simulink model "Hopf_AXILite"  (R2020a)
settings: Solver=VariableStepAuto  StartTime=0.0  StopTime=500  RelTol=1e-3
undefined symbols (not defined in the file): AXI4, Lite
libraries: xbsIndex_r4 x256
(part 2 of 2)

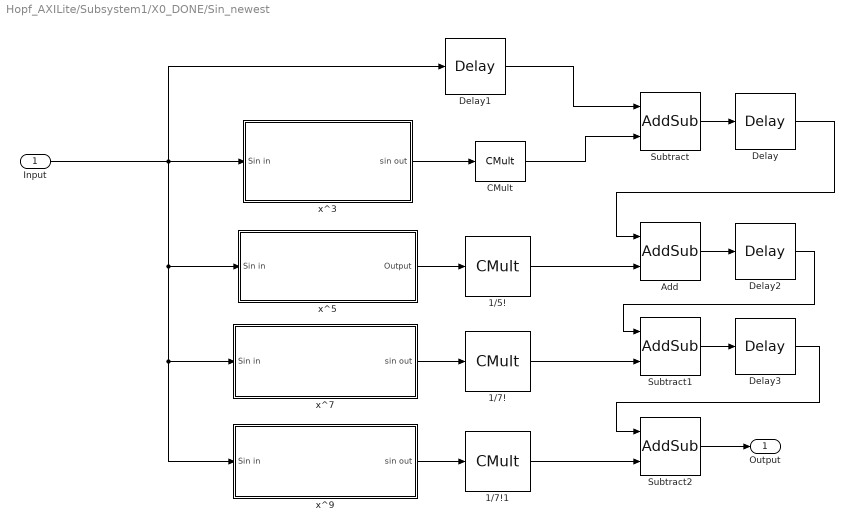
== system Hopf_AXILite/Subsystem1/X0_DONE/Sin_newest ==
  "Input " : Inport
  1/5! : xbsIndex_r4/CMult  const=1/(1*2*3*4*5)  gui_display_data_type=Fixed-point  const_n_bits=24  const_bin_pt=18  float_type=Single  exp_bits=8  fraction_bits=24  en=off  latency=1  precision=User Defined  arith_type="Signed  (2's comp)"  n_bits=24  bin_pt=18  quantization=Truncate  overflow=Wrap  use_behavioral_HDL=off  mem_type=Distributed RAM  pipeline=off  dbl_ovrd=off  block_type=cmult
  1/7! : xbsIndex_r4/CMult  const=1/(1*2*3*4*5*6*7)  gui_display_data_type=Fixed-point  const_n_bits=24  const_bin_pt=18  float_type=Single  exp_bits=8  fraction_bits=24  en=off  latency=1  precision=User Defined  arith_type="Signed  (2's comp)"  n_bits=24  bin_pt=18  quantization=Truncate  overflow=Wrap  use_behavioral_HDL=off  mem_type=Distributed RAM  pipeline=off  dbl_ovrd=off  block_type=cmult
  1/7!1 : xbsIndex_r4/CMult  const=1/(1*2*3*4*5*6*7*8*9)  gui_display_data_type=Fixed-point  const_n_bits=24  const_bin_pt=18  float_type=Single  exp_bits=8  fraction_bits=24  en=off  latency=1  precision=User Defined  arith_type="Signed  (2's comp)"  n_bits=24  bin_pt=18  quantization=Truncate  overflow=Wrap  use_behavioral_HDL=off  mem_type=Distributed RAM  pipeline=off  dbl_ovrd=off  block_type=cmult
  Add : xbsIndex_r4/AddSub  mode=Addition  use_carryin=off  use_carryout=off  en=off  latency=1  precision=User Defined  arith_type=Unsigned  n_bits=24  bin_pt=18  quantization=Truncate  overflow=Wrap  use_behavioral_HDL=off  hw_selection=Fabric  pipelined=off  dbl_ovrd=off  block_type=addsub
  CMult : xbsIndex_r4/CMult  const=1/2  gui_display_data_type=Fixed-point  const_n_bits=24  const_bin_pt=18  float_type=Single  exp_bits=8  fraction_bits=24  en=off  latency=1  precision=User Defined  arith_type="Signed  (2's comp)"  n_bits=24  bin_pt=19  quantization=Truncate  overflow=Wrap  use_behavioral_HDL=off  mem_type=Distributed RAM  pipeline=off  dbl_ovrd=off  block_type=cmult
  Delay : xbsIndex_r4/Delay  rst=off  infoeditControl=Selection of Reset will increase slice count due to use of real FFs and instead of SRLs  en=off  latency=2  reg_retiming=off  dbl_ovrd=off  block_type=delay
  Delay1 : xbsIndex_r4/Delay  rst=off  infoeditControl=Selection of Reset will increase slice count due to use of real FFs and instead of SRLs  en=off  latency=7  reg_retiming=off  dbl_ovrd=off  block_type=delay
  Delay2 : xbsIndex_r4/Delay  rst=off  infoeditControl=Selection of Reset will increase slice count due to use of real FFs and instead of SRLs  en=off  latency=2  reg_retiming=off  dbl_ovrd=off  block_type=delay
  Delay3 : xbsIndex_r4/Delay  rst=off  infoeditControl=Selection of Reset will increase slice count due to use of real FFs and instead of SRLs  en=off  latency=2  reg_retiming=off  dbl_ovrd=off  block_type=delay
  Subtract : xbsIndex_r4/AddSub  mode=Subtraction  use_carryin=off  use_carryout=off  en=off  latency=1  precision=User Defined  arith_type=Unsigned  n_bits=24  bin_pt=18  quantization=Truncate  overflow=Wrap  use_behavioral_HDL=off  hw_selection=Fabric  pipelined=off  dbl_ovrd=off  block_type=addsub
  Subtract1 : xbsIndex_r4/AddSub  mode=Subtraction  use_carryin=off  use_carryout=off  en=off  latency=1  precision=User Defined  arith_type=Unsigned  n_bits=24  bin_pt=18  quantization=Truncate  overflow=Wrap  use_behavioral_HDL=off  hw_selection=Fabric  pipelined=off  dbl_ovrd=off  block_type=addsub
  Subtract2 : xbsIndex_r4/AddSub  mode=Addition  use_carryin=off  use_carryout=off  en=off  latency=1  precision=User Defined  arith_type=Unsigned  n_bits=24  bin_pt=18  quantization=Truncate  overflow=Wrap  use_behavioral_HDL=off  hw_selection=Fabric  pipelined=off  dbl_ovrd=off  block_type=addsub
  x^3 : Subsystem
  x^5 : Subsystem
  x^7 : Subsystem
  x^9 : Subsystem
  Output : Outport
  wires:
  Add/1 -> Delay2/1
  Subtract1/1 -> Delay3/1
  1/5!/1 -> Add/2
  1/7!/1 -> Subtract1/2
  Delay1/1 -> Subtract/1
  "Input "/1 -> Delay1/1, x^3/1(Sin in), x^9/1(Sin in), x^7/1(Sin in), x^5/1(Sin in)
  x^3/1(sin out) -> CMult/1
  x^5/1(Output) -> 1/5!/1
  x^7/1(sin out) -> 1/7!/1
  Subtract/1 -> Delay/1
  Delay2/1 -> Subtract1/1
  x^9/1(sin out) -> 1/7!1/1
  Delay3/1 -> Subtract2/1
  1/7!1/1 -> Subtract2/2
  Subtract2/1 -> Output/1
  Delay/1 -> Add/1
  CMult/1 -> Subtract/2

== system Hopf_AXILite/Subsystem1/Calculation x1/Sin_newest/x^3 ==
  Sin in : Inport
  Mult2 : xbsIndex_r4/Mult  precision=User Defined  arith_type="Signed  (2's comp)"  n_bits=24  bin_pt=18  quantization=Truncate  overflow=Wrap  en=off  latency=3  use_behavioral_HDL=off  opt=Speed  use_embedded=on  optimum_pipeline=off  pipeline=on  dbl_ovrd=off  use_rpm=on  placement_style=Triangular  block_type=mult
  Mult3 : xbsIndex_r4/Mult  precision=User Defined  arith_type="Signed  (2's comp)"  n_bits=24  bin_pt=18  quantization=Truncate  overflow=Wrap  en=off  latency=3  use_behavioral_HDL=off  opt=Speed  use_embedded=on  optimum_pipeline=off  pipeline=on  dbl_ovrd=off  use_rpm=on  placement_style=Triangular  block_type=mult
  sin out : Outport
  wires:
  Mult2/1 -> Mult3/1
  Sin in/1 -> Mult2/1, Mult3/2, Mult2/2
  Mult3/1 -> sin out/1

== system Hopf_AXILite/Subsystem1/Calculation x1/Sin_newest/x^5 ==
  Sin in : Inport
  Mult2 : xbsIndex_r4/Mult  precision=User Defined  arith_type="Signed  (2's comp)"  n_bits=24  bin_pt=18  quantization=Truncate  overflow=Wrap  en=off  latency=3  use_behavioral_HDL=off  opt=Speed  use_embedded=on  optimum_pipeline=off  pipeline=on  dbl_ovrd=off  use_rpm=on  placement_style=Triangular  block_type=mult
  Mult3 : xbsIndex_r4/Mult  precision=User Defined  arith_type="Signed  (2's comp)"  n_bits=24  bin_pt=18  quantization=Truncate  overflow=Wrap  en=off  latency=3  use_behavioral_HDL=off  opt=Speed  use_embedded=on  optimum_pipeline=off  pipeline=on  dbl_ovrd=off  use_rpm=on  placement_style=Triangular  block_type=mult
  Mult4 : xbsIndex_r4/Mult  precision=User Defined  arith_type="Signed  (2's comp)"  n_bits=24  bin_pt=18  quantization=Truncate  overflow=Wrap  en=off  latency=3  use_behavioral_HDL=off  opt=Speed  use_embedded=on  optimum_pipeline=off  pipeline=on  dbl_ovrd=off  use_rpm=on  placement_style=Triangular  block_type=mult
  Output : Outport
  wires:
  Mult3/1 -> Mult4/1, Mult4/2
  Mult2/1 -> Mult3/1
  Sin in/1 -> Mult2/1, Mult3/2, Mult2/2
  Mult4/1 -> Output/1

== system Hopf_AXILite/Subsystem1/Calculation x1/Sin_newest/x^7 ==
  Sin in : Inport
  Mult{1..4} (4 alike) : xbsIndex_r4/Mult  precision=User Defined  arith_type="Signed  (2's comp)"  n_bits=24  bin_pt=18  quantization=Truncate  overflow=Wrap  en=off  latency=3  use_behavioral_HDL=off  opt=Speed  use_embedded=on  optimum_pipeline=off  pipeline=on  dbl_ovrd=off  use_rpm=on  placement_style=Triangular  block_type=mult
  sin out : Outport
  wires:
  Mult2/1 -> Mult3/1
  Mult3/1 -> Mult4/1, Mult4/2
  Mult4/1 -> Mult1/2, Mult1/1
  Sin in/1 -> Mult3/2, Mult2/2, Mult2/1
  Mult1/1 -> sin out/1

== system Hopf_AXILite/Subsystem1/Calculation x1/Sin_newest/x^9 ==
  Sin in : Inport
  Mult{1..5} (5 alike) : xbsIndex_r4/Mult  precision=User Defined  arith_type="Signed  (2's comp)"  n_bits=24  bin_pt=18  quantization=Truncate  overflow=Wrap  en=off  latency=3  use_behavioral_HDL=off  opt=Speed  use_embedded=on  optimum_pipeline=off  pipeline=on  dbl_ovrd=off  use_rpm=on  placement_style=Triangular  block_type=mult
  sin out : Outport
  wires:
  Mult2/1 -> Mult3/1
  Mult3/1 -> Mult4/1, Mult4/2
  Mult4/1 -> Mult1/2, Mult1/1
  Sin in/1 -> Mult3/2, Mult2/2, Mult2/1
  Mult1/1 -> Mult5/1, Mult5/2
  Mult5/1 -> sin out/1

== system Hopf_AXILite/Subsystem1/Calculation x1/Sin_newest1/x^3 ==
  Sin in : Inport
  Mult2 : xbsIndex_r4/Mult  precision=User Defined  arith_type="Signed  (2's comp)"  n_bits=24  bin_pt=18  quantization=Truncate  overflow=Wrap  en=off  latency=3  use_behavioral_HDL=off  opt=Speed  use_embedded=on  optimum_pipeline=off  pipeline=on  dbl_ovrd=off  use_rpm=on  placement_style=Triangular  block_type=mult
  Mult3 : xbsIndex_r4/Mult  precision=User Defined  arith_type="Signed  (2's comp)"  n_bits=24  bin_pt=18  quantization=Truncate  overflow=Wrap  en=off  latency=3  use_behavioral_HDL=off  opt=Speed  use_embedded=on  optimum_pipeline=off  pipeline=on  dbl_ovrd=off  use_rpm=on  placement_style=Triangular  block_type=mult
  sin out : Outport
  wires:
  Mult2/1 -> Mult3/1
  Sin in/1 -> Mult2/1, Mult3/2, Mult2/2
  Mult3/1 -> sin out/1

== system Hopf_AXILite/Subsystem1/Calculation x1/Sin_newest1/x^5 ==
  Sin in : Inport
  Mult2 : xbsIndex_r4/Mult  precision=User Defined  arith_type="Signed  (2's comp)"  n_bits=24  bin_pt=18  quantization=Truncate  overflow=Wrap  en=off  latency=3  use_behavioral_HDL=off  opt=Speed  use_embedded=on  optimum_pipeline=off  pipeline=on  dbl_ovrd=off  use_rpm=on  placement_style=Triangular  block_type=mult
  Mult3 : xbsIndex_r4/Mult  precision=User Defined  arith_type="Signed  (2's comp)"  n_bits=24  bin_pt=18  quantization=Truncate  overflow=Wrap  en=off  latency=3  use_behavioral_HDL=off  opt=Speed  use_embedded=on  optimum_pipeline=off  pipeline=on  dbl_ovrd=off  use_rpm=on  placement_style=Triangular  block_type=mult
  Mult4 : xbsIndex_r4/Mult  precision=User Defined  arith_type="Signed  (2's comp)"  n_bits=24  bin_pt=18  quantization=Truncate  overflow=Wrap  en=off  latency=3  use_behavioral_HDL=off  opt=Speed  use_embedded=on  optimum_pipeline=off  pipeline=on  dbl_ovrd=off  use_rpm=on  placement_style=Triangular  block_type=mult
  Output : Outport
  wires:
  Mult3/1 -> Mult4/1, Mult4/2
  Mult2/1 -> Mult3/1
  Sin in/1 -> Mult2/1, Mult3/2, Mult2/2
  Mult4/1 -> Output/1

== system Hopf_AXILite/Subsystem1/Calculation x1/Sin_newest1/x^7 ==
  Sin in : Inport
  Mult{1..4} (4 alike) : xbsIndex_r4/Mult  precision=User Defined  arith_type="Signed  (2's comp)"  n_bits=24  bin_pt=18  quantization=Truncate  overflow=Wrap  en=off  latency=3  use_behavioral_HDL=off  opt=Speed  use_embedded=on  optimum_pipeline=off  pipeline=on  dbl_ovrd=off  use_rpm=on  placement_style=Triangular  block_type=mult
  sin out : Outport
  wires:
  Mult2/1 -> Mult3/1
  Mult3/1 -> Mult4/1, Mult4/2
  Mult4/1 -> Mult1/2, Mult1/1
  Sin in/1 -> Mult3/2, Mult2/2, Mult2/1
  Mult1/1 -> sin out/1

== system Hopf_AXILite/Subsystem1/Calculation x1/Sin_newest1/x^9 ==
  Sin in : Inport
  Mult{1..5} (5 alike) : xbsIndex_r4/Mult  precision=User Defined  arith_type="Signed  (2's comp)"  n_bits=24  bin_pt=18  quantization=Truncate  overflow=Wrap  en=off  latency=3  use_behavioral_HDL=off  opt=Speed  use_embedded=on  optimum_pipeline=off  pipeline=on  dbl_ovrd=off  use_rpm=on  placement_style=Triangular  block_type=mult
  sin out : Outport
  wires:
  Mult2/1 -> Mult3/1
  Mult3/1 -> Mult4/1, Mult4/2
  Mult4/1 -> Mult1/2, Mult1/1
  Sin in/1 -> Mult3/2, Mult2/2, Mult2/1
  Mult1/1 -> Mult5/1, Mult5/2
  Mult5/1 -> sin out/1

== system Hopf_AXILite/Subsystem1/Calculation x2/Cosine_newest/POW 10 ==
  Input : Inport
  Mult{1..5} (5 alike) : xbsIndex_r4/Mult  precision=User Defined  arith_type="Signed  (2's comp)"  n_bits=24  bin_pt=18  quantization=Truncate  overflow=Wrap  en=off  latency=3  use_behavioral_HDL=off  opt=Speed  use_embedded=on  optimum_pipeline=off  pipeline=on  dbl_ovrd=off  use_rpm=on  placement_style=Triangular  block_type=mult
  ^10 : Outport
  wires:
  Mult2/1 -> Mult1/1, Mult1/2
  Mult1/1 -> Mult3/1, Mult3/2
  Mult3/1 -> Mult4/1, Mult4/2
  Mult4/1 -> Mult5/1, Mult5/2
  Input/1 -> Mult2/1, Mult2/2
  Mult5/1 -> ^10/1

== system Hopf_AXILite/Subsystem1/Calculation x2/Cosine_newest/POW 8 ==
  Input : Inport
  Mult{1..4} (4 alike) : xbsIndex_r4/Mult  precision=User Defined  arith_type="Signed  (2's comp)"  n_bits=24  bin_pt=18  quantization=Truncate  overflow=Wrap  en=off  latency=3  use_behavioral_HDL=off  opt=Speed  use_embedded=on  optimum_pipeline=off  pipeline=on  dbl_ovrd=off  use_rpm=on  placement_style=Triangular  block_type=mult
  ^8 : Outport
  wires:
  Mult2/1 -> Mult1/1, Mult1/2
  Mult1/1 -> Mult3/1, Mult3/2
  Mult3/1 -> Mult4/1, Mult4/2
  Input/1 -> Mult2/1, Mult2/2
  Mult4/1 -> ^8/1

== system Hopf_AXILite/Subsystem1/Calculation x2/Cosine_newest/Subsystem ==
  Input : Inport
  Mult1 : xbsIndex_r4/Mult  precision=User Defined  arith_type="Signed  (2's comp)"  n_bits=24  bin_pt=18  quantization=Truncate  overflow=Wrap  en=off  latency=3  use_behavioral_HDL=off  opt=Speed  use_embedded=on  optimum_pipeline=off  pipeline=on  dbl_ovrd=off  use_rpm=on  placement_style=Triangular  block_type=mult
  Mult2 : xbsIndex_r4/Mult  precision=User Defined  arith_type="Signed  (2's comp)"  n_bits=24  bin_pt=18  quantization=Truncate  overflow=Wrap  en=off  latency=3  use_behavioral_HDL=off  opt=Speed  use_embedded=on  optimum_pipeline=off  pipeline=on  dbl_ovrd=off  use_rpm=on  placement_style=Triangular  block_type=mult
  ^4 : Outport
  wires:
  Mult2/1 -> Mult1/2, Mult1/1
  Input/1 -> Mult2/2, Mult2/1
  Mult1/1 -> ^4/1

== system Hopf_AXILite/Subsystem1/Calculation x2/Cosine_newest/Subsystem1 ==
  Input : Inport
  Mult1 : xbsIndex_r4/Mult  precision=User Defined  arith_type="Signed  (2's comp)"  n_bits=24  bin_pt=18  quantization=Truncate  overflow=Wrap  en=off  latency=3  use_behavioral_HDL=off  opt=Speed  use_embedded=on  optimum_pipeline=off  pipeline=on  dbl_ovrd=off  use_rpm=on  placement_style=Triangular  block_type=mult
  Mult2 : xbsIndex_r4/Mult  precision=User Defined  arith_type="Signed  (2's comp)"  n_bits=24  bin_pt=18  quantization=Truncate  overflow=Wrap  en=off  latency=3  use_behavioral_HDL=off  opt=Speed  use_embedded=on  optimum_pipeline=off  pipeline=on  dbl_ovrd=off  use_rpm=on  placement_style=Triangular  block_type=mult
  Mult3 : xbsIndex_r4/Mult  precision=User Defined  arith_type="Signed  (2's comp)"  n_bits=24  bin_pt=18  quantization=Truncate  overflow=Wrap  en=off  latency=3  use_behavioral_HDL=off  opt=Speed  use_embedded=on  optimum_pipeline=off  pipeline=on  dbl_ovrd=off  use_rpm=on  placement_style=Triangular  block_type=mult
  ^6 : Outport
  wires:
  Mult2/1 -> Mult1/2, Mult1/1
  Mult1/1 -> Mult3/2, Mult3/1
  Input/1 -> Mult2/2, Mult2/1
  Mult3/1 -> ^6/1

== system Hopf_AXILite/Subsystem1/Calculation x2/Cosine_newest1/POW 10 ==
  Input : Inport
  Mult{1..5} (5 alike) : xbsIndex_r4/Mult  precision=User Defined  arith_type="Signed  (2's comp)"  n_bits=24  bin_pt=18  quantization=Truncate  overflow=Wrap  en=off  latency=3  use_behavioral_HDL=off  opt=Speed  use_embedded=on  optimum_pipeline=off  pipeline=on  dbl_ovrd=off  use_rpm=on  placement_style=Triangular  block_type=mult
  ^10 : Outport
  wires:
  Mult2/1 -> Mult1/1, Mult1/2
  Mult1/1 -> Mult3/1, Mult3/2
  Mult3/1 -> Mult4/1, Mult4/2
  Mult4/1 -> Mult5/1, Mult5/2
  Input/1 -> Mult2/1, Mult2/2
  Mult5/1 -> ^10/1

== system Hopf_AXILite/Subsystem1/Calculation x2/Cosine_newest1/POW 8 ==
  Input : Inport
  Mult{1..4} (4 alike) : xbsIndex_r4/Mult  precision=User Defined  arith_type="Signed  (2's comp)"  n_bits=24  bin_pt=18  quantization=Truncate  overflow=Wrap  en=off  latency=3  use_behavioral_HDL=off  opt=Speed  use_embedded=on  optimum_pipeline=off  pipeline=on  dbl_ovrd=off  use_rpm=on  placement_style=Triangular  block_type=mult
  ^8 : Outport
  wires:
  Mult2/1 -> Mult1/1, Mult1/2
  Mult1/1 -> Mult3/1, Mult3/2
  Mult3/1 -> Mult4/1, Mult4/2
  Input/1 -> Mult2/1, Mult2/2
  Mult4/1 -> ^8/1

== system Hopf_AXILite/Subsystem1/Calculation x2/Cosine_newest1/Subsystem ==
  Input : Inport
  Mult1 : xbsIndex_r4/Mult  precision=User Defined  arith_type="Signed  (2's comp)"  n_bits=24  bin_pt=18  quantization=Truncate  overflow=Wrap  en=off  latency=3  use_behavioral_HDL=off  opt=Speed  use_embedded=on  optimum_pipeline=off  pipeline=on  dbl_ovrd=off  use_rpm=on  placement_style=Triangular  block_type=mult
  Mult2 : xbsIndex_r4/Mult  precision=User Defined  arith_type="Signed  (2's comp)"  n_bits=24  bin_pt=18  quantization=Truncate  overflow=Wrap  en=off  latency=3  use_behavioral_HDL=off  opt=Speed  use_embedded=on  optimum_pipeline=off  pipeline=on  dbl_ovrd=off  use_rpm=on  placement_style=Triangular  block_type=mult
  ^4 : Outport
  wires:
  Mult2/1 -> Mult1/2, Mult1/1
  Input/1 -> Mult2/2, Mult2/1
  Mult1/1 -> ^4/1

== system Hopf_AXILite/Subsystem1/Calculation x2/Cosine_newest1/Subsystem1 ==
  Input : Inport
  Mult1 : xbsIndex_r4/Mult  precision=User Defined  arith_type="Signed  (2's comp)"  n_bits=24  bin_pt=18  quantization=Truncate  overflow=Wrap  en=off  latency=3  use_behavioral_HDL=off  opt=Speed  use_embedded=on  optimum_pipeline=off  pipeline=on  dbl_ovrd=off  use_rpm=on  placement_style=Triangular  block_type=mult
  Mult2 : xbsIndex_r4/Mult  precision=User Defined  arith_type="Signed  (2's comp)"  n_bits=24  bin_pt=18  quantization=Truncate  overflow=Wrap  en=off  latency=3  use_behavioral_HDL=off  opt=Speed  use_embedded=on  optimum_pipeline=off  pipeline=on  dbl_ovrd=off  use_rpm=on  placement_style=Triangular  block_type=mult
  Mult3 : xbsIndex_r4/Mult  precision=User Defined  arith_type="Signed  (2's comp)"  n_bits=24  bin_pt=18  quantization=Truncate  overflow=Wrap  en=off  latency=3  use_behavioral_HDL=off  opt=Speed  use_embedded=on  optimum_pipeline=off  pipeline=on  dbl_ovrd=off  use_rpm=on  placement_style=Triangular  block_type=mult
  ^6 : Outport
  wires:
  Mult2/1 -> Mult1/2, Mult1/1
  Mult1/1 -> Mult3/2, Mult3/1
  Input/1 -> Mult2/2, Mult2/1
  Mult3/1 -> ^6/1

== system Hopf_AXILite/Subsystem1/Calculation x3/Cosine_newest/POW 10 ==
  Input : Inport
  Mult{1..5} (5 alike) : xbsIndex_r4/Mult  precision=User Defined  arith_type="Signed  (2's comp)"  n_bits=24  bin_pt=18  quantization=Truncate  overflow=Wrap  en=off  latency=3  use_behavioral_HDL=off  opt=Speed  use_embedded=on  optimum_pipeline=off  pipeline=on  dbl_ovrd=off  use_rpm=on  placement_style=Triangular  block_type=mult
  ^10 : Outport
  wires:
  Mult2/1 -> Mult1/1, Mult1/2
  Mult1/1 -> Mult3/1, Mult3/2
  Mult3/1 -> Mult4/1, Mult4/2
  Mult4/1 -> Mult5/1, Mult5/2
  Input/1 -> Mult2/1, Mult2/2
  Mult5/1 -> ^10/1

== system Hopf_AXILite/Subsystem1/Calculation x3/Cosine_newest/POW 8 ==
  Input : Inport
  Mult{1..4} (4 alike) : xbsIndex_r4/Mult  precision=User Defined  arith_type="Signed  (2's comp)"  n_bits=24  bin_pt=18  quantization=Truncate  overflow=Wrap  en=off  latency=3  use_behavioral_HDL=off  opt=Speed  use_embedded=on  optimum_pipeline=off  pipeline=on  dbl_ovrd=off  use_rpm=on  placement_style=Triangular  block_type=mult
  ^8 : Outport
  wires:
  Mult2/1 -> Mult1/1, Mult1/2
  Mult1/1 -> Mult3/1, Mult3/2
  Mult3/1 -> Mult4/1, Mult4/2
  Input/1 -> Mult2/1, Mult2/2
  Mult4/1 -> ^8/1

== system Hopf_AXILite/Subsystem1/Calculation x3/Cosine_newest/Subsystem ==
  Input : Inport
  Mult1 : xbsIndex_r4/Mult  precision=User Defined  arith_type="Signed  (2's comp)"  n_bits=24  bin_pt=18  quantization=Truncate  overflow=Wrap  en=off  latency=3  use_behavioral_HDL=off  opt=Speed  use_embedded=on  optimum_pipeline=off  pipeline=on  dbl_ovrd=off  use_rpm=on  placement_style=Triangular  block_type=mult
  Mult2 : xbsIndex_r4/Mult  precision=User Defined  arith_type="Signed  (2's comp)"  n_bits=24  bin_pt=18  quantization=Truncate  overflow=Wrap  en=off  latency=3  use_behavioral_HDL=off  opt=Speed  use_embedded=on  optimum_pipeline=off  pipeline=on  dbl_ovrd=off  use_rpm=on  placement_style=Triangular  block_type=mult
  ^4 : Outport
  wires:
  Mult2/1 -> Mult1/2, Mult1/1
  Input/1 -> Mult2/2, Mult2/1
  Mult1/1 -> ^4/1

== system Hopf_AXILite/Subsystem1/Calculation x3/Cosine_newest/Subsystem1 ==
  Input : Inport
  Mult1 : xbsIndex_r4/Mult  precision=User Defined  arith_type="Signed  (2's comp)"  n_bits=24  bin_pt=18  quantization=Truncate  overflow=Wrap  en=off  latency=3  use_behavioral_HDL=off  opt=Speed  use_embedded=on  optimum_pipeline=off  pipeline=on  dbl_ovrd=off  use_rpm=on  placement_style=Triangular  block_type=mult
  Mult2 : xbsIndex_r4/Mult  precision=User Defined  arith_type="Signed  (2's comp)"  n_bits=24  bin_pt=18  quantization=Truncate  overflow=Wrap  en=off  latency=3  use_behavioral_HDL=off  opt=Speed  use_embedded=on  optimum_pipeline=off  pipeline=on  dbl_ovrd=off  use_rpm=on  placement_style=Triangular  block_type=mult
  Mult3 : xbsIndex_r4/Mult  precision=User Defined  arith_type="Signed  (2's comp)"  n_bits=24  bin_pt=18  quantization=Truncate  overflow=Wrap  en=off  latency=3  use_behavioral_HDL=off  opt=Speed  use_embedded=on  optimum_pipeline=off  pipeline=on  dbl_ovrd=off  use_rpm=on  placement_style=Triangular  block_type=mult
  ^6 : Outport
  wires:
  Mult2/1 -> Mult1/2, Mult1/1
  Mult1/1 -> Mult3/2, Mult3/1
  Input/1 -> Mult2/2, Mult2/1
  Mult3/1 -> ^6/1

== system Hopf_AXILite/Subsystem1/Calculation x3/Sin_newest/x^3 ==
  Sin in : Inport
  Mult2 : xbsIndex_r4/Mult  precision=User Defined  arith_type="Signed  (2's comp)"  n_bits=24  bin_pt=18  quantization=Truncate  overflow=Wrap  en=off  latency=3  use_behavioral_HDL=off  opt=Speed  use_embedded=on  optimum_pipeline=off  pipeline=on  dbl_ovrd=off  use_rpm=on  placement_style=Triangular  block_type=mult
  Mult3 : xbsIndex_r4/Mult  precision=User Defined  arith_type="Signed  (2's comp)"  n_bits=24  bin_pt=18  quantization=Truncate  overflow=Wrap  en=off  latency=3  use_behavioral_HDL=off  opt=Speed  use_embedded=on  optimum_pipeline=off  pipeline=on  dbl_ovrd=off  use_rpm=on  placement_style=Triangular  block_type=mult
  sin out : Outport
  wires:
  Mult2/1 -> Mult3/1
  Sin in/1 -> Mult2/1, Mult3/2, Mult2/2
  Mult3/1 -> sin out/1

== system Hopf_AXILite/Subsystem1/Calculation x3/Sin_newest/x^5 ==
  Sin in : Inport
  Mult2 : xbsIndex_r4/Mult  precision=User Defined  arith_type="Signed  (2's comp)"  n_bits=24  bin_pt=18  quantization=Truncate  overflow=Wrap  en=off  latency=3  use_behavioral_HDL=off  opt=Speed  use_embedded=on  optimum_pipeline=off  pipeline=on  dbl_ovrd=off  use_rpm=on  placement_style=Triangular  block_type=mult
  Mult3 : xbsIndex_r4/Mult  precision=User Defined  arith_type="Signed  (2's comp)"  n_bits=24  bin_pt=18  quantization=Truncate  overflow=Wrap  en=off  latency=3  use_behavioral_HDL=off  opt=Speed  use_embedded=on  optimum_pipeline=off  pipeline=on  dbl_ovrd=off  use_rpm=on  placement_style=Triangular  block_type=mult
  Mult4 : xbsIndex_r4/Mult  precision=User Defined  arith_type="Signed  (2's comp)"  n_bits=24  bin_pt=18  quantization=Truncate  overflow=Wrap  en=off  latency=3  use_behavioral_HDL=off  opt=Speed  use_embedded=on  optimum_pipeline=off  pipeline=on  dbl_ovrd=off  use_rpm=on  placement_style=Triangular  block_type=mult
  Output : Outport
  wires:
  Mult3/1 -> Mult4/1, Mult4/2
  Mult2/1 -> Mult3/1
  Sin in/1 -> Mult2/1, Mult3/2, Mult2/2
  Mult4/1 -> Output/1

== system Hopf_AXILite/Subsystem1/Calculation x3/Sin_newest/x^7 ==
  Sin in : Inport
  Mult{1..4} (4 alike) : xbsIndex_r4/Mult  precision=User Defined  arith_type="Signed  (2's comp)"  n_bits=24  bin_pt=18  quantization=Truncate  overflow=Wrap  en=off  latency=3  use_behavioral_HDL=off  opt=Speed  use_embedded=on  optimum_pipeline=off  pipeline=on  dbl_ovrd=off  use_rpm=on  placement_style=Triangular  block_type=mult
  sin out : Outport
  wires:
  Mult2/1 -> Mult3/1
  Mult3/1 -> Mult4/1, Mult4/2
  Mult4/1 -> Mult1/2, Mult1/1
  Sin in/1 -> Mult3/2, Mult2/2, Mult2/1
  Mult1/1 -> sin out/1

== system Hopf_AXILite/Subsystem1/Calculation x3/Sin_newest/x^9 ==
  Sin in : Inport
  Mult{1..5} (5 alike) : xbsIndex_r4/Mult  precision=User Defined  arith_type="Signed  (2's comp)"  n_bits=24  bin_pt=18  quantization=Truncate  overflow=Wrap  en=off  latency=3  use_behavioral_HDL=off  opt=Speed  use_embedded=on  optimum_pipeline=off  pipeline=on  dbl_ovrd=off  use_rpm=on  placement_style=Triangular  block_type=mult
  sin out : Outport
  wires:
  Mult2/1 -> Mult3/1
  Mult3/1 -> Mult4/1, Mult4/2
  Mult4/1 -> Mult1/2, Mult1/1
  Sin in/1 -> Mult3/2, Mult2/2, Mult2/1
  Mult1/1 -> Mult5/1, Mult5/2
  Mult5/1 -> sin out/1

== system Hopf_AXILite/Subsystem1/X0_DONE/Cosine_newest/POW 10 ==
  Input : Inport
  Mult{1..5} (5 alike) : xbsIndex_r4/Mult  precision=User Defined  arith_type="Signed  (2's comp)"  n_bits=24  bin_pt=18  quantization=Truncate  overflow=Wrap  en=off  latency=3  use_behavioral_HDL=off  opt=Speed  use_embedded=on  optimum_pipeline=off  pipeline=on  dbl_ovrd=off  use_rpm=on  placement_style=Triangular  block_type=mult
  ^10 : Outport
  wires:
  Mult2/1 -> Mult1/1, Mult1/2
  Mult1/1 -> Mult3/1, Mult3/2
  Mult3/1 -> Mult4/1, Mult4/2
  Mult4/1 -> Mult5/1, Mult5/2
  Input/1 -> Mult2/1, Mult2/2
  Mult5/1 -> ^10/1

== system Hopf_AXILite/Subsystem1/X0_DONE/Cosine_newest/POW 8 ==
  Input : Inport
  Mult{1..4} (4 alike) : xbsIndex_r4/Mult  precision=User Defined  arith_type="Signed  (2's comp)"  n_bits=24  bin_pt=18  quantization=Truncate  overflow=Wrap  en=off  latency=3  use_behavioral_HDL=off  opt=Speed  use_embedded=on  optimum_pipeline=off  pipeline=on  dbl_ovrd=off  use_rpm=on  placement_style=Triangular  block_type=mult
  ^8 : Outport
  wires:
  Mult2/1 -> Mult1/1, Mult1/2
  Mult1/1 -> Mult3/1, Mult3/2
  Mult3/1 -> Mult4/1, Mult4/2
  Input/1 -> Mult2/1, Mult2/2
  Mult4/1 -> ^8/1

== system Hopf_AXILite/Subsystem1/X0_DONE/Cosine_newest/Subsystem ==
  Input : Inport
  Mult1 : xbsIndex_r4/Mult  precision=User Defined  arith_type="Signed  (2's comp)"  n_bits=24  bin_pt=18  quantization=Truncate  overflow=Wrap  en=off  latency=3  use_behavioral_HDL=off  opt=Speed  use_embedded=on  optimum_pipeline=off  pipeline=on  dbl_ovrd=off  use_rpm=on  placement_style=Triangular  block_type=mult
  Mult2 : xbsIndex_r4/Mult  precision=User Defined  arith_type="Signed  (2's comp)"  n_bits=24  bin_pt=18  quantization=Truncate  overflow=Wrap  en=off  latency=3  use_behavioral_HDL=off  opt=Speed  use_embedded=on  optimum_pipeline=off  pipeline=on  dbl_ovrd=off  use_rpm=on  placement_style=Triangular  block_type=mult
  ^4 : Outport
  wires:
  Mult2/1 -> Mult1/2, Mult1/1
  Input/1 -> Mult2/2, Mult2/1
  Mult1/1 -> ^4/1

== system Hopf_AXILite/Subsystem1/X0_DONE/Cosine_newest/Subsystem1 ==
  Input : Inport
  Mult1 : xbsIndex_r4/Mult  precision=User Defined  arith_type="Signed  (2's comp)"  n_bits=24  bin_pt=18  quantization=Truncate  overflow=Wrap  en=off  latency=3  use_behavioral_HDL=off  opt=Speed  use_embedded=on  optimum_pipeline=off  pipeline=on  dbl_ovrd=off  use_rpm=on  placement_style=Triangular  block_type=mult
  Mult2 : xbsIndex_r4/Mult  precision=User Defined  arith_type="Signed  (2's comp)"  n_bits=24  bin_pt=18  quantization=Truncate  overflow=Wrap  en=off  latency=3  use_behavioral_HDL=off  opt=Speed  use_embedded=on  optimum_pipeline=off  pipeline=on  dbl_ovrd=off  use_rpm=on  placement_style=Triangular  block_type=mult
  Mult3 : xbsIndex_r4/Mult  precision=User Defined  arith_type="Signed  (2's comp)"  n_bits=24  bin_pt=18  quantization=Truncate  overflow=Wrap  en=off  latency=3  use_behavioral_HDL=off  opt=Speed  use_embedded=on  optimum_pipeline=off  pipeline=on  dbl_ovrd=off  use_rpm=on  placement_style=Triangular  block_type=mult
  ^6 : Outport
  wires:
  Mult2/1 -> Mult1/2, Mult1/1
  Mult1/1 -> Mult3/2, Mult3/1
  Input/1 -> Mult2/2, Mult2/1
  Mult3/1 -> ^6/1

== system Hopf_AXILite/Subsystem1/X0_DONE/Sin_newest/x^3 ==
  Sin in : Inport
  Mult2 : xbsIndex_r4/Mult  precision=User Defined  arith_type="Signed  (2's comp)"  n_bits=24  bin_pt=18  quantization=Truncate  overflow=Wrap  en=off  latency=3  use_behavioral_HDL=off  opt=Speed  use_embedded=on  optimum_pipeline=off  pipeline=on  dbl_ovrd=off  use_rpm=on  placement_style=Triangular  block_type=mult
  Mult3 : xbsIndex_r4/Mult  precision=User Defined  arith_type="Signed  (2's comp)"  n_bits=24  bin_pt=18  quantization=Truncate  overflow=Wrap  en=off  latency=3  use_behavioral_HDL=off  opt=Speed  use_embedded=on  optimum_pipeline=off  pipeline=on  dbl_ovrd=off  use_rpm=on  placement_style=Triangular  block_type=mult
  sin out : Outport
  wires:
  Mult2/1 -> Mult3/1
  Sin in/1 -> Mult2/1, Mult3/2, Mult2/2
  Mult3/1 -> sin out/1

== system Hopf_AXILite/Subsystem1/X0_DONE/Sin_newest/x^5 ==
  Sin in : Inport
  Mult2 : xbsIndex_r4/Mult  precision=User Defined  arith_type="Signed  (2's comp)"  n_bits=24  bin_pt=18  quantization=Truncate  overflow=Wrap  en=off  latency=3  use_behavioral_HDL=off  opt=Speed  use_embedded=on  optimum_pipeline=off  pipeline=on  dbl_ovrd=off  use_rpm=on  placement_style=Triangular  block_type=mult
  Mult3 : xbsIndex_r4/Mult  precision=User Defined  arith_type="Signed  (2's comp)"  n_bits=24  bin_pt=18  quantization=Truncate  overflow=Wrap  en=off  latency=3  use_behavioral_HDL=off  opt=Speed  use_embedded=on  optimum_pipeline=off  pipeline=on  dbl_ovrd=off  use_rpm=on  placement_style=Triangular  block_type=mult
  Mult4 : xbsIndex_r4/Mult  precision=User Defined  arith_type="Signed  (2's comp)"  n_bits=24  bin_pt=18  quantization=Truncate  overflow=Wrap  en=off  latency=3  use_behavioral_HDL=off  opt=Speed  use_embedded=on  optimum_pipeline=off  pipeline=on  dbl_ovrd=off  use_rpm=on  placement_style=Triangular  block_type=mult
  Output : Outport
  wires:
  Mult3/1 -> Mult4/1, Mult4/2
  Mult2/1 -> Mult3/1
  Sin in/1 -> Mult2/1, Mult3/2, Mult2/2
  Mult4/1 -> Output/1

== system Hopf_AXILite/Subsystem1/X0_DONE/Sin_newest/x^7 ==
  Sin in : Inport
  Mult{1..4} (4 alike) : xbsIndex_r4/Mult  precision=User Defined  arith_type="Signed  (2's comp)"  n_bits=24  bin_pt=18  quantization=Truncate  overflow=Wrap  en=off  latency=3  use_behavioral_HDL=off  opt=Speed  use_embedded=on  optimum_pipeline=off  pipeline=on  dbl_ovrd=off  use_rpm=on  placement_style=Triangular  block_type=mult
  sin out : Outport
  wires:
  Mult2/1 -> Mult3/1
  Mult3/1 -> Mult4/1, Mult4/2
  Mult4/1 -> Mult1/2, Mult1/1
  Sin in/1 -> Mult3/2, Mult2/2, Mult2/1
  Mult1/1 -> sin out/1

== system Hopf_AXILite/Subsystem1/X0_DONE/Sin_newest/x^9 ==
  Sin in : Inport
  Mult{1..5} (5 alike) : xbsIndex_r4/Mult  precision=User Defined  arith_type="Signed  (2's comp)"  n_bits=24  bin_pt=18  quantization=Truncate  overflow=Wrap  en=off  latency=3  use_behavioral_HDL=off  opt=Speed  use_embedded=on  optimum_pipeline=off  pipeline=on  dbl_ovrd=off  use_rpm=on  placement_style=Triangular  block_type=mult
  sin out : Outport
  wires:
  Mult2/1 -> Mult3/1
  Mult3/1 -> Mult4/1, Mult4/2
  Mult4/1 -> Mult1/2, Mult1/1
  Sin in/1 -> Mult3/2, Mult2/2, Mult2/1
  Mult1/1 -> Mult5/1, Mult5/2
  Mult5/1 -> sin out/1
